simulink model "VehRT_211219"  (R2019b)
settings: Solver=ode5  StartTime=0.0  StopTime=Inf  FixedStep=Ts  RelTol=1e-3  EnableMultiTasking=on
InitFcn:
  | VehRT_Init_211219;
  | Ts=0.0005;
values from neighbouring files (symbols this model uses):
  damping_p = 0.113    [VehRT_Init_211219.m]
  Ff_ab_p = 0.41    [VehRT_Init_211219.m]
  Ff_c_p = 0.4    [VehRT_Init_211219.m]
  friction_enable = 1    [VehRT_Init_211219.m]
  sigma0_p = 200    [VehRT_Init_211219.m]
  sigma1_p = (200)^0.5    (= 14.1421356237)    [VehRT_Init_211219.m]
  td = 0.01    [VehRT_Init_211219.m]
  theta_sb_p = 0.03    [VehRT_Init_211219.m]
undefined symbols (not defined in the file or in its folder): C, canChannel, D, DiscIntNeverNeededParam, g, IO306, Kf, Kr, Lf, Lr, M, magnitude, sigma, trajectory_x11_, trajectory_x12_, trajectory_x13_, trajectory_x14_, trajectory_x15_, trajectory_x16_, trajectory_x17_, trajectory_x21_, trajectory_x22_, trajectory_x23_, trajectory_x24_, trajectory_x25_, trajectory_x26_, trajectory_x27_, trajectory_y11_, trajectory_y12_, trajectory_y13_, trajectory_y14_, trajectory_y15_, trajectory_y16_, trajectory_y17_, trajectory_y21_, trajectory_y22_, trajectory_y23_, trajectory_y24_, trajectory_y25_, trajectory_y26_, trajectory_y27_, zeta
libraries: canmsglib x31, speedgoatlib_IO612 x20, slrtlib x15, simulink x5, speedgoatlib_IO133 x3, xpcutilitieslib x2, canlib x2, xpcrtudplib x2, speedgoatlib_fpga x1, speedgoatlib_fpga_dio x1, autolibshared x1, speedgoatlib_fpga_quadrature x1
(part 1 of 4)
settings Model: SimulationMode=external  Creator=CECLAB  LastModifiedBy=CECLAB
settings SolverCC: ConcurrentTasks=on  AutoInsertRateTranBlk=on  InsertRTBMode=Never (minimum delay)
settings DataIOCC: SaveFormat=StructureWithTime  SaveOutput=off  SignalLogging=off  DSMLogging=off  ReturnWorkspaceOutputs=off
settings OptimizationCC: BlockReduction=off  OptimizeBlockIOStorage=off  BufferReuse=off  GlobalBufferReuse=off  ExpressionFolding=off  LocalBlockOutputs=off  OptimizeDataStoreBuffers=off  BusAssignmentInplaceUpdate=off
settings DebuggingCC: ArithmeticOperatorsInVariantConditions=warning
settings HardwareCC: ProdBitPerPointer=32  ProdBitPerSizeT=32  ProdBitPerPtrDiffT=32  ProdLargestAtomicFloat=None  ProdWordSize=32  ProdLongLongMode=on  ProdHWDeviceType=Generic->32-bit x86 compatible
settings SFSimCC: SimUseLocalCustomCode=off  CustomCodeUndefinedFunction=UseInterfaceOnly
settings RTWCC: Description=Simulink Real-Time  SystemTargetFile=slrt.tlc  TemplateMakefile=slrt_default_tmf  RTWUseLocalCustomCode=off  CodeExecutionProfiling=on  RTWCompilerOptimization=on
settings SimulinkRealTimeCC: SupportVariableSizeSignals=on  PreserveStateflowLocalDataDimensions=off  RL32LogTETModifier=off  xPCConcurrentTasks=on

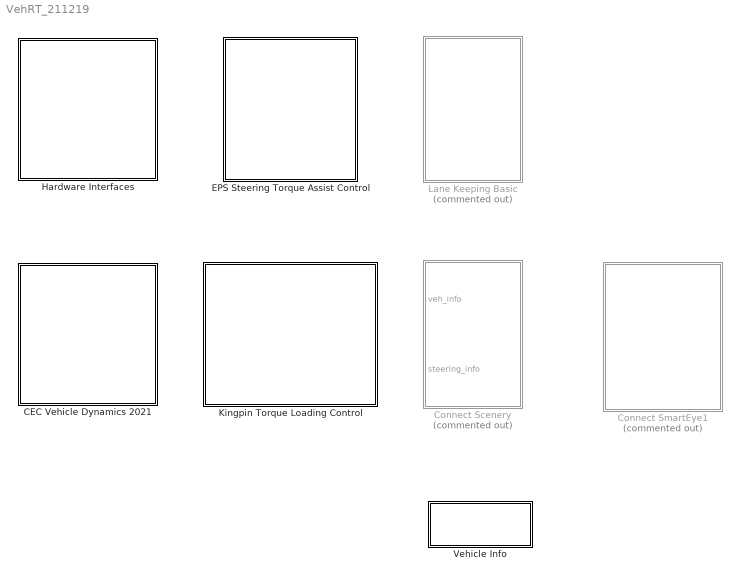
== system VehRT_211219 ==
  CEC Vehicle Dynamics 2021 : Subsystem
  Connect Scenery : Subsystem  Commented=on
  Connect SmartEye1 : Subsystem  Commented=on
  EPS Steering Torque Assist Control : Subsystem
  Hardware Interfaces : Subsystem
  Kingpin Torque Loading Control : Subsystem
  Lane Keeping Basic : Subsystem  Commented=on
  Vehicle Info : Subsystem

== system VehRT_211219/CEC Vehicle Dynamics 2021 ==
  note: CEC Vehicle Dynamics 2021
  Bus Selector : BusSelector  OutputSignals=str_Mpinion,veh_Vx
  CEC Vehicle Model 2021 : Subsystem  SystemSampleTime=0.001
      mask Display:
      | pos = get_param(gcb, 'Position');
      | width = pos(3) - pos(1);
      | height = pos(4) - pos(2);
      | p = min(width, height);
      | qx = (width-p)/2;
      | qy = (height-p)/2;
      | plt_body = [0.504672897196262,0.795560747663551;0.586448598130841,0.870327102803738;0.626168224299065,0.882009345794393;0.684579439252337,0.877336448598131;0.745327102803738,0.842289719626168;0.817757009345794,0.786214953271028;0.871495327102804,0.706775700934579;0.887850467289720,0.676401869158879;0.890186915887851,0.629672897196262;0.878504672897196,0.580607476635514;0.869158878504673,0.564252336448598;0.773364485981309,0.473130841121495;0.778037383177570,0.421728971962617;0.775700934579439,0.407710280373832;0.761682242990654,0.393691588785047;0.747663551401869,0.393691588785047;0.735981308411215,0.431074766355140;0.455607476635514,0.155373831775701;0.401869158878505,0.113317757009346;0.352803738317757,0.0852803738317758;0.313084112149533,0.0876168224299065;0.273364485981308,0.0992990654205608;0.207943925233645,0.160046728971963;0.149532710280374,0.220794392523365;0.107476635514019,0.267523364485981;0.0957943925233645,0.318925233644860;0.0981308411214953,0.358644859813084;0.121495327102804,0.400700934579439;0.441588785046729,0.730140186915888;0.404205607476636,0.732476635514019;0.397196261682243,0.741822429906542;0.401869158878505,0.760514018691589;0.422897196261682,0.769859813084112;0.453271028037383,0.762850467289720;0.478971962616822,0.762850467289720;0.504672897196262,0.795560747663551];
      | plt_body2 = [0.492990654205608,0.744158878504673;0.530373831775701,0.718457943925234;0.593457943925234,0.669392523364486;0.637850467289720,0.622663551401869;0.689252336448598,0.568925233644860;0.719626168224299,0.526869158878505;0.747663551401869,0.484813084112150;0.630841121495327,0.445093457943925;0.457943925233645,0.620327102803738;0.455607476635514,0.632009345794393;0.492990654205608,0.744158878504673];
      | plt_body3 = [0.635514018691589,0.424065420560748;0.740654205607477,0.461448598130841;0.448598130841122,0.176401869158878;0.469626168224299,0.255841121495327;0.635514018691589,0.424065420560748];
      | plt_body4 = [0.271028037383178,0.445093457943925;0.450934579439252,0.265186915887851;0.432242990654206,0.176401869158878;0.429906542056075,0.174065420560748;0.348130841121495,0.244158878504673;0.250000000000000,0.342289719626168;0.179906542056075,0.421728971962617;0.184579439252337,0.424065420560748;0.271028037383178,0.445093457943925]; %;0.186915887850467,0.447429906542056
      | plt_body5 = [0.266355140186916,0.463785046728972;0.184579439252337,0.445093457943925;0.469626168224299,0.727803738317757;0.432242990654206,0.620327102803738;0.266355140186916,0.463785046728972];
      | plt_body6 = [0.600467289719626,0.858644859813084;0.635514018691589,0.870327102803738;0.661214953271028,0.865654205607477;0.647196261682243,0.851635514018692;0.619158878504673,0.849299065420561;0.600467289719626,0.858644859813084];
      | plt_body7 = [0.866822429906542,0.596962616822430;0.857476635514019,0.610981308411215;0.862149532710280,0.636682242990654;0.871495327102804,0.655373831775701;0.871495327102804,0.657710280373832;0.876168224299065,0.632009345794393;0.871495327102804,0.594626168224299;0.866822429906542,0.596962616822430];
      | plt_body8 = [0.630841121495327,0.258177570093458;0.700934579439252,0.274532710280374;0.703271028037383,0.239485981308411;0.651869158878505,0.237149532710280;0.651869158878505,0.157710280373832;0.698598130841122,0.141355140186916;0.700934579439252,0.108644859813084;0.628504672897196,0.141355140186916;0.630841121495327,0.258177570093458];
      | plt_body9 = [0.710280373831776,0.272196261682243;0.707943925233645,0.113317757009346;0.785046728971963,0.132009345794393;0.785046728971963,0.155373831775701;0.742990654205608,0.150700934579439;0.740654205607477,0.178738317757009;0.785046728971963,0.185747663551402;0.787383177570094,0.206775700934579;0.742990654205608,0.209112149532710;0.740654205607477,0.241822429906542;0.785046728971963,0.234813084112150;0.785046728971963,0.260514018691589;0.710280373831776,0.272196261682243];
      | plt_body10 = [0.794392523364486,0.260514018691589;0.796728971962617,0.129672897196262;0.880841121495327,0.110981308411215;0.880841121495327,0.146028037383178;0.822429906542056,0.155373831775701;0.820093457943925,0.237149532710280;0.878504672897196,0.244158878504673;0.878504672897196,0.276869158878505;0.794392523364486,0.260514018691589];
      | plot([0,1,1,0]*width,[0,0,1,1]*height)
      | plot(plt_body(:,1)*p+qx,plt_body(:,2)*p+qy);
      | plot(plt_body2(:,1)*p+qx,plt_body2(:,2)*p+qy);
      | plot(plt_body3(:,1)*p+qx,plt_body3(:,2)*p+qy);
      | plot(plt_body4(:,1)*p+qx,plt_body4(:,2)*p+qy);
      | plot(plt_body5(:,1)*p+qx,plt_body5(:,2)*p+qy);
      | plot(plt_body6(:,1)*p+qx,plt_body6(:,2)*p+qy);
      | plot(plt_body7(:,1)*p+qx,plt_body7(:,2)*p+qy);
      | plot(plt_body8(:,1)*p+qx,plt_body8(:,2)*p+qy);
      | plot(plt_body9(:,1)*p+qx,plt_body9(:,2)*p+qy);
      | plot(plt_body10(:,1)*p+qx,plt_body10(:,2)*p+qy);
  Gain : Gain  Gain=0.01
  Gain1 : Gain  Gain=0.01
  Reset with Clutch : Subsystem
  manual_driving : Constant  Value=0
  mu_test : Subsystem
  zero_speed : Constant  Value=0
  tag scope: Veh_info=global, Vehicle_speed=global, pinion_torque=global
  wires:
  [pinion_angle] -> CEC Vehicle Model 2021/1(sta)
  [pedal_acc] -> Gain/1
  [pedal_brk] -> Gain1/1
  mu_test/1(mus) -> CEC Vehicle Model 2021/4(mu_road)
  zero_speed/1 -> CEC Vehicle Model 2021/5(spd_target)
  manual_driving/1 -> CEC Vehicle Model 2021/6(acc_mode)
  Reset with Clutch/1(rst) -> CEC Vehicle Model 2021/7(reset)
  CEC Vehicle Model 2021/1(Info) -> Bus Selector/1, [Veh_info]
  Bus Selector/1 -> [pinion_torque]  "<str_Mpinion>"
  Bus Selector/2 -> [Vehicle_speed]  "<veh_Vx>"
  Gain1/1 -> CEC Vehicle Model 2021/3(brk_m)
  Gain/1 -> CEC Vehicle Model 2021/2(thr_m)

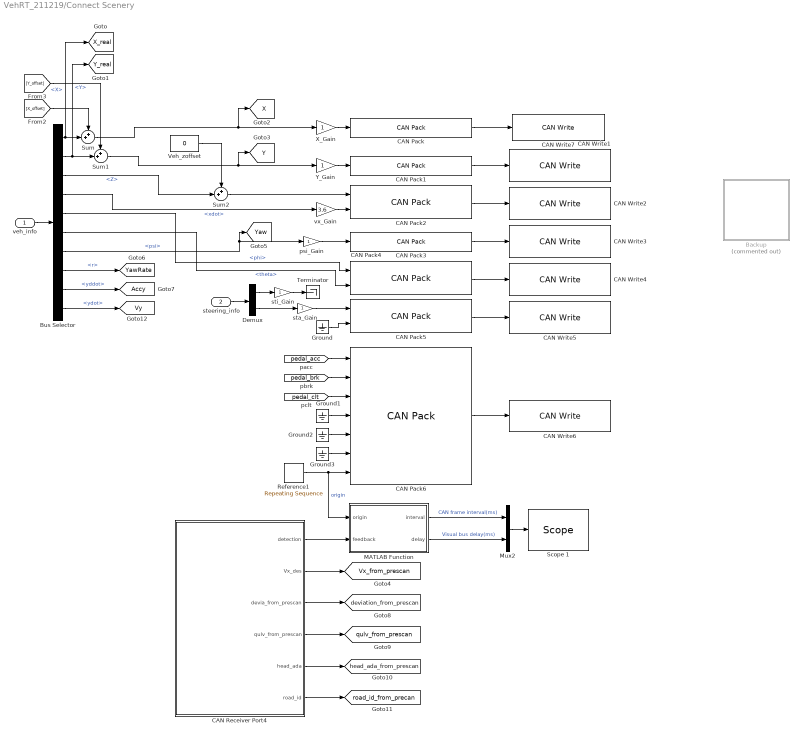
== system VehRT_211219/Connect Scenery ==
  veh_info : Inport
  steering_info : Inport  Port=2
  Backup : Subsystem  Commented=on
  Bus Selector : BusSelector  OutputSignals=InertFrm.Cg.Disp.X,InertFrm.Cg.Disp.Y,InertFrm.Cg.Disp.Z,BdyFrm.Cg.Vel.xdot,InertFrm.Cg.Ang.phi,InertFrm.Cg.Ang.theta,InertFrm.Cg.Ang.psi,BdyFrm.Cg.AngVel.r,BdyFrm.Cg.Acc.yddot,BdyFrm.Cg.Vel.ydot
  CAN Pack : canmsglib/CAN Pack  MsgList=(none)  MsgName=CAN Msg  MsgIDType=Standard (11-bit identifier)  MsgIdentifier=100  MsgLength=8  Remote=off  ApplyMinMax=off  BusOutput=off  SignalInfo={ 'x', '0', '64', 'LE', 'double', 'Standard', '0', '1', '0', '-Inf', 'Inf' }
      settings: SourceProductName=Vehicle Network Toolbox  SourceProductBaseCode=VN  DataFormat=manually specified signals
  CAN Pack1 : canmsglib/CAN Pack  MsgList=(none)  MsgName=CAN Msg  MsgIDType=Standard (11-bit identifier)  MsgIdentifier=101  MsgLength=8  Remote=off  ApplyMinMax=off  BusOutput=off  SignalInfo={ 'y', '0', '64', 'LE', 'double', 'Standard', '0', '1', '0', '-Inf', 'Inf' }
      settings: SourceProductName=Vehicle Network Toolbox  SourceProductBaseCode=VN  DataFormat=manually specified signals
  CAN Pack2 : canmsglib/CAN Pack  MsgList=(none)  MsgName=CAN Msg  MsgIDType=Standard (11-bit identifier)  MsgIdentifier=102  MsgLength=8  Remote=off  ApplyMinMax=off  BusOutput=off  SignalInfo={ 'z', '0', '32', 'LE', 'single', 'Standard', '0', '1', '0', '-Inf', 'Inf'; 'vx', '32', '32', 'LE', 'single', 'Standard', '0', '1', '0', '-Inf', 'Inf' }
      settings: SourceProductName=Vehicle Network Toolbox  SourceProductBaseCode=VN  DataFormat=manually specified signals
  CAN Pack3 : canmsglib/CAN Pack  MsgList=(none)  MsgName=CAN Msg  MsgIDType=Standard (11-bit identifier)  MsgIdentifier=103  MsgLength=8  Remote=off  ApplyMinMax=off  BusOutput=off  SignalInfo={ 'yaw', '0', '64', 'LE', 'double', 'Standard', '0', '1', '0', '-Inf', 'Inf' }
      settings: SourceProductName=Vehicle Network Toolbox  SourceProductBaseCode=VN  DataFormat=manually specified signals
  CAN Pack4 : canmsglib/CAN Pack  MsgList=(none)  MsgName=CAN Msg  MsgIDType=Standard (11-bit identifier)  MsgIdentifier=104  MsgLength=8  Remote=off  ApplyMinMax=off  BusOutput=off  SignalInfo={ 'roll', '0', '32', 'LE', 'single', 'Standard', '0', '1', '0', '-Inf', 'Inf'; 'pitch', '32', '32', 'LE', 'single', 'Standard', '0', '1', '0', '-Inf', 'Inf' }
      settings: SourceProductName=Vehicle Network Toolbox  SourceProductBaseCode=VN  DataFormat=manually specified signals
  CAN Pack5 : canmsglib/CAN Pack  MsgList=(none)  MsgName=CAN Msg  MsgIDType=Standard (11-bit identifier)  MsgIdentifier=105  MsgLength=8  Remote=off  ApplyMinMax=off  BusOutput=off  SignalInfo={ 'sta', '0', '32', 'LE', 'single', 'Standard', '0', '1', '0', '-Inf', 'Inf'; 'reserved', '32', '32', 'LE', 'single', 'Standard', '0', '1', '0', '-Inf', 'Inf' }
      settings: SourceProductName=Vehicle Network Toolbox  SourceProductBaseCode=VN  DataFormat=manually specified signals
  CAN Pack6 : canmsglib/CAN Pack  MsgList=(none)  MsgName=CAN Msg  MsgIDType=Standard (11-bit identifier)  MsgIdentifier=106  MsgLength=8  Remote=off  ApplyMinMax=off  BusOutput=off  SignalInfo={ 'pedal_acc', '0', '8', 'LE', 'unsigned', 'Standard', '0', '1', '0', '-Inf', 'Inf'; 'pedal_brk', '8', '8', 'LE', 'unsigned', 'Standard', '0', '1', '0', '-Inf', 'Inf'; 'pedal_clt', '16', '8', 'LE', 'unsigned', 'Standard', '0', '1', '0', '-Inf', 'Inf'; 'sw1', '24', '8', 'LE', 'unsigned', 'Standard', '0', '1', '0', '-Inf', 'Inf'; 'sw2', '32', '8', 'LE', 'unsigned', 'Standard', '0', '1', '0', '-Inf', 'Inf'; 'sw3', '40', '8', 'LE', 'unsigned', 'Standard', '0', '1', '0', '-Inf', 'Inf'; 'test', '48', '16', 'LE', 'unsigned', 'Standard', '0', '1', '0', '-Inf', 'Inf' }
      settings: SourceProductName=Vehicle Network Toolbox  SourceProductBaseCode=VN  DataFormat=manually specified signals
  CAN Receiver Port4 : Subsystem  TreatAsAtomicUnit=on
  CAN Write{1..7} (7 alike) : speedgoatlib_IO612/CAN Write  id=1  sampleTime=0.005  portSelection=2  messageType=CAN  enaStatusPort=off  protl=IO612  ptIdx=1  isFDMod=0
      settings: SourceProductName=Simulink Real-Time: Speedgoat Library
  Demux : Demux  Outputs=2
  Ground{,1..3} (4 alike) : Ground
  MATLAB Function : MATLAB Function  TreatAsAtomicUnit=on  SystemSampleTime=0.001
  Mux2 : Mux  Inputs=2
  Reference1 : simulink/Sources/Repeating Sequence  rep_seq_t=[0 2]  rep_seq_y=[0 65535]
  Scope 1 : slrtlib/Displays and Logging/Scope   scopeno=14  scopetype=Target  autostart=on  viewmode=Graphical sliding  formatstr='%15.6f'  grid=on  ylimits=[0,200]  nosamples=4000  noprepostsamples=0  interleave=1  triggermode=FreeRun  triggersignal=1  trigsignalfromport=off  triggerlevel=0.0  triggerslope=Either  triggerscope=1  triggersample=0  filename=data.dat  mode=Lazy  writesize=512  autorestart=off  dynamicfilemode=off  maxwritefilesize=512*1024^2
  Sum : Sum  Inputs=++|
  Sum1 : Sum  Inputs=++|
  Sum2 : Sum  Inputs=++|
  Terminator : Terminator
  Veh_zoffset : Constant  Value=0
  X_Gain : Gain
  Y_Gain : Gain
  psi_Gain : Gain
  sta_Gain : Gain
  sti_Gain : Gain
  "vx_Gain " : Gain  Gain=3.6
  tag scope: Accy=global, Vx_from_prescan=global, Vy=global, X=global, X_real=global, Y=global, Y_real=global, Yaw=global, YawRate=global, deviation_from_prescan=global, head_ada_from_prescan=global, qulv_from_prescan=global, road_id_from_precan=global
  wires:
  sta_Gain/1 -> CAN Pack5/1
  Demux/1 -> sti_Gain/1
  sti_Gain/1 -> Terminator/1
  Bus Selector/7 -> [Yaw], psi_Gain/1  "<psi>"
  Bus Selector/1 -> [X_real], Sum/2  "<X>"
  Bus Selector/3 -> Sum2/2  "<Z>"
  Bus Selector/2 -> [Y_real], Sum1/2  "<Y>"
  veh_info/1 -> Bus Selector/1
  steering_info/1 -> Demux/1
  Demux/2 -> sta_Gain/1
  MATLAB Function/2(delay) -> Mux2/2  "Visual bus delay(ms)"
  Mux2/1 -> Scope 1/1
  MATLAB Function/1(interval) -> Mux2/1  "CAN frame interval(ms)"
  Sum/1 -> [X], X_Gain/1
  Sum1/1 -> [Y], Y_Gain/1
  [X_offset] -> Sum/1
  [Y_offset] -> Sum1/1
  Bus Selector/4 -> "vx_Gain "/1  "<xdot>"
  "vx_Gain "/1 -> CAN Pack2/2
  Bus Selector/5 -> CAN Pack4/1  "<phi>"
  Bus Selector/6 -> CAN Pack4/2  "<theta>"
  X_Gain/1 -> CAN Pack/1
  Y_Gain/1 -> CAN Pack1/1
  Ground/1 -> CAN Pack5/2
  [pedal_acc] -> CAN Pack6/1
  [pedal_brk] -> CAN Pack6/2
  [pedal_clt] -> CAN Pack6/3
  Ground1/1 -> CAN Pack6/4
  Ground2/1 -> CAN Pack6/5
  Ground3/1 -> CAN Pack6/6
  Reference1/1 -> CAN Pack6/7, MATLAB Function/1(origin)  "origin"
  CAN Receiver Port4/1(detection) -> MATLAB Function/2(feedback)
  CAN Receiver Port4/2(Vx_des) -> [Vx_from_prescan]
  Sum2/1 -> CAN Pack2/1
  Veh_zoffset/1 -> Sum2/1
  Bus Selector/8 -> [YawRate]  "<r>"
  Bus Selector/9 -> [Accy]  "<yddot>"
  CAN Receiver Port4/3(devia_from_prescan) -> [deviation_from_prescan]
  CAN Receiver Port4/4(qulv_from_prescan) -> [qulv_from_prescan]
  CAN Receiver Port4/5(head_ada) -> [head_ada_from_prescan]
  psi_Gain/1 -> CAN Pack3/1
  CAN Receiver Port4/6(road_id) -> [road_id_from_precan]
  Bus Selector/10 -> [Vy]  "<ydot>"
  CAN Pack/1 -> CAN Write7/1
  CAN Pack6/1 -> CAN Write6/1
  CAN Pack1/1 -> CAN Write1/1
  CAN Pack2/1 -> CAN Write2/1
  CAN Pack3/1 -> CAN Write3/1
  CAN Pack4/1 -> CAN Write4/1
  CAN Pack5/1 -> CAN Write5/1

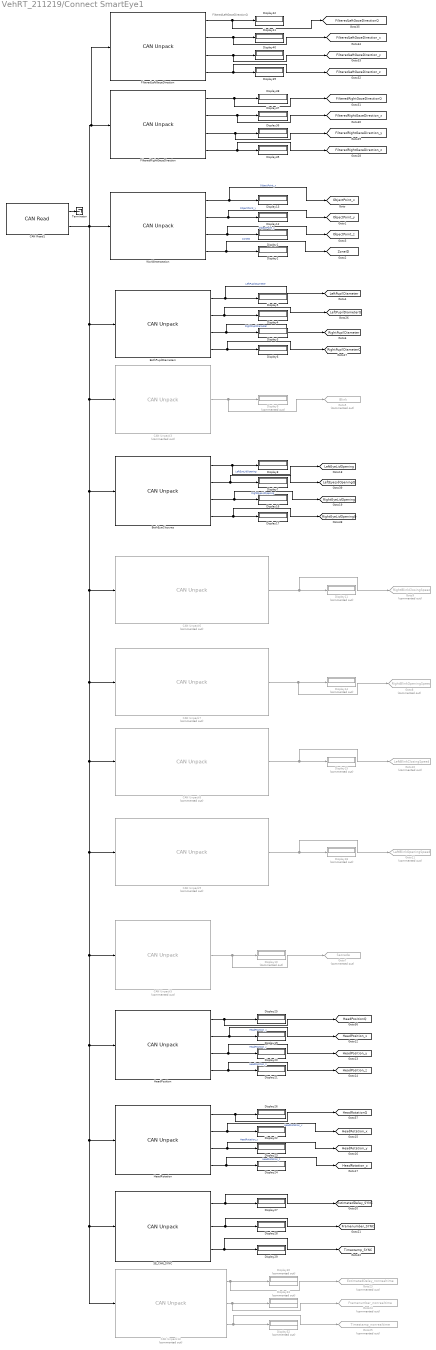
== system VehRT_211219/Connect SmartEye1 ==
  note: FilteredLeftGazeDirectionQ
  BothEyeClosures : canmsglib/CAN Unpack  CANdbFile=D:\Simulink\chenjiachen\realtime\smarteye.dbc  MsgList=SE_CAN_BOTHEYECLOSURES  MsgName=SE_CAN_BOTHEYECLOSURES  MsgIDType=Standard (11-bit identifier)  MsgIdentifier=1032  MsgLength=8  SignalInfo={'LeftEyeLidOpening','0','16','LE','signed','Standard','0','0.1','0','-3276.8','3276.7';'LeftEyeLidOpeningQ','16','16','LE','unsigned','Standard','0','0.0001','0','0','1';'RightEyeLidOpening','32','16','LE','signed','Standard','0','0.1','0','-3276.8','3276.7';'RightEyeLidOpeningQ','48','16','LE','unsigned','Standard','0','0.0001','0','0','1'}  IDPort=off  TimestampPort=off  ErrorPort=off  RemotePort=off  LengthPort=off  StatusPort=off  ApplyMinMax=off
      settings: SourceProductName=Simulink Real-Time  DataFormat=CANdb specified signals
  BothPupilDiameters : canmsglib/CAN Unpack  CANdbFile=D:\Simulink\chenjiachen\realtime\smarteye.dbc  MsgList=SE_CAN_BOTHPUPILDIAMETERS  MsgName=SE_CAN_BOTHPUPILDIAMETERS  MsgIDType=Standard (11-bit identifier)  MsgIdentifier=1034  MsgLength=8  SignalInfo={'LeftPupilDiameter','0','16','LE','signed','Standard','0','0.1','0','-3276.8','3276.7';'LeftPupilDiameterQ','16','16','LE','unsigned','Standard','0','0.0001','0','0','1';'RightPupilDiameter','32','16','LE','signed','Standard','0','0.1','0','-3276.8','3276.7';'RightPupilDiameterQ','48','16','LE','unsigned','Standard','0','0.0001','0','0','1'}  IDPort=off  TimestampPort=off  ErrorPort=off  RemotePort=off  LengthPort=off  StatusPort=off  ApplyMinMax=off
      settings: SourceProductName=Simulink Real-Time  DataFormat=CANdb specified signals
  CAN Read1 : speedgoatlib_IO612/CAN Read  id=1  sampleTime=-1  portSelection=3  messageType=CAN  protl=IO612  ptIdx=2  isFDMod=0
      settings: SourceProductName=Simulink Real-Time: Speedgoat Library
  CAN Unpack13 : canmsglib/CAN Unpack  Commented=on  CANdbFile=D:\Simulink\chenjiachen\realtime\smarteye.dbc  MsgList=SE_CAN_SYNCH_NON_REALTIME  MsgName=SE_CAN_SYNCH_NON_REALTIME  MsgIDType=Standard (11-bit identifier)  MsgIdentifier=1040  MsgLength=8  SignalInfo={'EstimatedDelay','48','16','LE','unsigned','Standard','0','0.1','0','0','6553.5';'Framenumber','0','32','LE','unsigned','Standard','0','1','0','0','4294967295';'Timestamp','32','16','LE','unsigned','Standard','0','0.1','0','0','6553.5'}  IDPort=off  TimestampPort=off  ErrorPort=off  RemotePort=off  LengthPort=off  StatusPort=off  ApplyMinMax=off
      settings: SourceProductName=Simulink Real-Time  DataFormat=CANdb specified signals
  CAN Unpack3 : canmsglib/CAN Unpack  Commented=on  CANdbFile=D:\Simulink\chenjiachen\realtime\smarteye.dbc  MsgList=SE_CAN_BLINK  MsgName=SE_CAN_BLINK  MsgIDType=Standard (11-bit identifier)  MsgIdentifier=1042  MsgLength=4  SignalInfo={'Blink','0','32','LE','unsigned','Standard','0','1','0','0','1'}  IDPort=off  TimestampPort=off  ErrorPort=off  RemotePort=off  LengthPort=off  StatusPort=off  ApplyMinMax=off
      settings: SourceProductName=Simulink Real-Time  DataFormat=CANdb specified signals
  CAN Unpack5 : canmsglib/CAN Unpack  Commented=on  CANdbFile=D:\Simulink\chenjiachen\realtime\smarteye.dbc  MsgList=SE_CAN_SACCADE  MsgName=SE_CAN_SACCADE  MsgIDType=Standard (11-bit identifier)  MsgIdentifier=1043  MsgLength=4  SignalInfo={'Saccade','0','32','LE','unsigned','Standard','0','1','0','0','1'}  IDPort=off  TimestampPort=off  ErrorPort=off  RemotePort=off  LengthPort=off  StatusPort=off  ApplyMinMax=off
      settings: SourceProductName=Simulink Real-Time  DataFormat=CANdb specified signals
  CAN Unpack6 : canmsglib/CAN Unpack  Commented=on  CANdbFile=D:\Simulink\chenjiachen\realtime\smarteye.dbc  MsgList=SE_CAN_RIGHTBLINKCLOSINGSPEED  MsgName=SE_CAN_RIGHTBLINKCLOSINGSPEED  MsgIDType=Standard (11-bit identifier)  MsgIdentifier=1052  MsgLength=2  SignalInfo={'RightBlinkClosingSpeed','0','16','LE','signed','Standard','0','0.0001','0','-3.2768','3.2767'}  IDPort=off  TimestampPort=off  ErrorPort=off  RemotePort=off  LengthPort=off  StatusPort=off  ApplyMinMax=off
      settings: SourceProductName=Simulink Real-Time  DataFormat=CANdb specified signals
  CAN Unpack7 : canmsglib/CAN Unpack  Commented=on  CANdbFile=D:\Simulink\chenjiachen\realtime\smarteye.dbc  MsgList=SE_CAN_RIGHTBLINKOPENINGSPEED  MsgName=SE_CAN_RIGHTBLINKOPENINGSPEED  MsgIDType=Standard (11-bit identifier)  MsgIdentifier=1055  MsgLength=2  SignalInfo={'RightBlinkOpeningSpeed','0','16','LE','signed','Standard','0','0.0001','0','-3.2768','3.2767'}  IDPort=off  TimestampPort=off  ErrorPort=off  RemotePort=off  LengthPort=off  StatusPort=off  ApplyMinMax=off
      settings: SourceProductName=Simulink Real-Time  DataFormat=CANdb specified signals
  CAN Unpack8 : canmsglib/CAN Unpack  Commented=on  CANdbFile=D:\Simulink\chenjiachen\realtime\smarteye.dbc  MsgList=SE_CAN_LEFTBLINKCLOSINGSPEED  MsgName=SE_CAN_LEFTBLINKCLOSINGSPEED  MsgIDType=Standard (11-bit identifier)  MsgIdentifier=1046  MsgLength=2  SignalInfo={'LeftBlinkClosingSpeed','0','16','LE','signed','Standard','0','0.0001','0','-3.2768','3.2767'}  IDPort=off  TimestampPort=off  ErrorPort=off  RemotePort=off  LengthPort=off  StatusPort=off  ApplyMinMax=off
      settings: SourceProductName=Simulink Real-Time  DataFormat=CANdb specified signals
  CAN Unpack9 : canmsglib/CAN Unpack  Commented=on  CANdbFile=D:\Simulink\chenjiachen\realtime\smarteye.dbc  MsgList=SE_CAN_LEFTBLINKOPENINGSPEED  MsgName=SE_CAN_LEFTBLINKOPENINGSPEED  MsgIDType=Standard (11-bit identifier)  MsgIdentifier=1049  MsgLength=2  SignalInfo={'LeftBlinkOpeningSpeed','0','16','LE','signed','Standard','0','0.0001','0','-3.2768','3.2767'}  IDPort=off  TimestampPort=off  ErrorPort=off  RemotePort=off  LengthPort=off  StatusPort=off  ApplyMinMax=off
      settings: SourceProductName=Simulink Real-Time  DataFormat=CANdb specified signals
  Display{1..8,12..13,16..17,19..29,35..42} (31 alike) : Display
  Display{9..11,14..15,18,30,32..33} (9 alike) : Display  Commented=on
  FilteredLeftGazeDirection : canmsglib/CAN Unpack  CANdbFile=D:\Simulink\chenjiachen\realtime\smarteye.dbc  MsgList=SE_CAN_FILTEREDLEFTGAZEDIRECTION  MsgName=SE_CAN_FILTEREDLEFTGAZEDIRECTION  MsgIDType=Standard (11-bit identifier)  MsgIdentifier=1038  MsgLength=8  SignalInfo={'FilteredLeftGazeDirectionQ','48','16','LE','unsigned','Standard','0','0.0001','0','0','1';'FilteredLeftGazeDirection_x','0','16','LE','signed','Standard','0','0.0001','0','-1','1';'FilteredLeftGazeDirection_y','16','16','LE','signed','Standard','0','0.0001','0','-1','1';'FilteredLeftGazeDirection_z','32','16','LE','signed','Standard','0','0.0001','0','-1','1'}  IDPort=off  TimestampPort=off  ErrorPort=off  RemotePort=off  LengthPort=off  StatusPort=off  ApplyMinMax=off
      settings: SourceProductName=Simulink Real-Time  DataFormat=CANdb specified signals
  FilteredRightGazeDirection : canmsglib/CAN Unpack  CANdbFile=D:\Simulink\chenjiachen\realtime\smarteye.dbc  MsgList=SE_CAN_FILTEREDRIGHTGAZEDIRECTION  MsgName=SE_CAN_FILTEREDRIGHTGAZEDIRECTION  MsgIDType=Standard (11-bit identifier)  MsgIdentifier=1039  MsgLength=8  SignalInfo={'FilteredRightGazeDirectionQ','48','16','LE','unsigned','Standard','0','0.0001','0','0','1';'FilteredRightGazeDirection_x','0','16','LE','signed','Standard','0','0.0001','0','-1','1';'FilteredRightGazeDirection_y','16','16','LE','signed','Standard','0','0.0001','0','-1','1';'FilteredRightGazeDirection_z','32','16','LE','signed','Standard','0','0.0001','0','-1','1'}  IDPort=off  TimestampPort=off  ErrorPort=off  RemotePort=off  LengthPort=off  StatusPort=off  ApplyMinMax=off
      settings: SourceProductName=Simulink Real-Time  DataFormat=CANdb specified signals
  Goto10 : Goto  Commented=on  GotoTag=LeftBlinkClosingSpeed  TagVisibility=global
  Goto11 : Goto  Commented=on  GotoTag=LeftBlinkOpeningSpeed  TagVisibility=global
  Goto23 : Goto  Commented=on  GotoTag=EstimatedDelay_nonrealtime  TagVisibility=global
  Goto24 : Goto  Commented=on  GotoTag=Framenumber_nonrealtime  TagVisibility=global
  Goto25 : Goto  Commented=on  GotoTag=Timestamp_nonrealtime  TagVisibility=global
  Goto5 : Goto  Commented=on  GotoTag=Blink  TagVisibility=global
  Goto7 : Goto  Commented=on  GotoTag=Saccade  TagVisibility=global
  Goto8 : Goto  Commented=on  GotoTag=RightBlinkOpeningSpeed  TagVisibility=global
  Goto9 : Goto  Commented=on  GotoTag=RightBlinkClosingSpeed  TagVisibility=global
  HeadPosition : canmsglib/CAN Unpack  CANdbFile=D:\Simulink\chenjiachen\realtime\smarteye.dbc  MsgList=SE_CAN_HEADPOSITION  MsgName=SE_CAN_HEADPOSITION  MsgIDType=Standard (11-bit identifier)  MsgIdentifier=1027  MsgLength=8  SignalInfo={'HeadPositionQ','48','16','LE','unsigned','Standard','0','0.0001','0','0','1';'HeadPosition_x','0','16','LE','signed','Standard','0','0.1','0','-3276.8','3276.7';'HeadPosition_y','16','16','LE','signed','Standard','0','0.1','0','-3276.8','3276.7';'HeadPosition_z','32','16','LE','signed','Standard','0','0.1','0','-3276.8','3276.7'}  IDPort=off  TimestampPort=off  ErrorPort=off  RemotePort=off  LengthPort=off  StatusPort=off  ApplyMinMax=off
      settings: SourceProductName=Simulink Real-Time  DataFormat=CANdb specified signals
  HeadRotation : canmsglib/CAN Unpack  CANdbFile=D:\Simulink\chenjiachen\realtime\smarteye.dbc  MsgList=SE_CAN_HEADROTATION  MsgName=SE_CAN_HEADROTATION  MsgIDType=Standard (11-bit identifier)  MsgIdentifier=1028  MsgLength=8  SignalInfo={'HeadRotationQ','48','16','LE','unsigned','Standard','0','0.0001','0','0','1';'HeadRotation_x','0','16','LE','signed','Standard','0','0.0001','0','-3.2768','3.2767';'HeadRotation_y','16','16','LE','signed','Standard','0','0.0001','0','-3.2768','3.2767';'HeadRotation_z','32','16','LE','signed','Standard','0','0.0001','0','-3.2768','3.2767'}  IDPort=off  TimestampPort=off  ErrorPort=off  RemotePort=off  LengthPort=off  StatusPort=off  ApplyMinMax=off
      settings: SourceProductName=Simulink Real-Time  DataFormat=CANdb specified signals
  SE_CAN_SYNC : canmsglib/CAN Unpack  CANdbFile=D:\Simulink\chenjiachen\realtime\smarteye.dbc  MsgList=SE_CAN_SYNC  MsgName=SE_CAN_SYNC  MsgIDType=Standard (11-bit identifier)  MsgIdentifier=1025  MsgLength=8  SignalInfo={'EstimatedDelay','48','16','LE','unsigned','Standard','0','0.1','0','0','6553.5';'Framenumber','0','32','LE','unsigned','Standard','0','1','0','0','4294967295';'Timestamp','32','16','LE','unsigned','Standard','0','0.1','0','0','6553.5'}  IDPort=off  TimestampPort=off  ErrorPort=off  RemotePort=off  LengthPort=off  StatusPort=off  ApplyMinMax=off
      settings: SourceProductName=Simulink Real-Time  DataFormat=CANdb specified signals
  Terminator : Terminator
  WorldIntersection : canmsglib/CAN Unpack  CANdbFile=D:\Simulink\chenjiachen\realtime\smarteye.dbc  MsgList=SE_CAN_WORLDINTERSECTION  MsgName=SE_CAN_WORLDINTERSECTION  MsgIDType=Standard (11-bit identifier)  MsgIdentifier=1036  MsgLength=8  SignalInfo={'ObjectPoint_x','16','16','LE','signed','Standard','0','0.1','0','-3276.8','3276.7';'ObjectPoint_y','32','16','LE','signed','Standard','0','0.1','0','-3276.8','3276.7';'ObjectPoint_z','48','16','LE','signed','Standard','0','0.1','0','-3276.8','3276.7';'ZoneID','0','16','LE','unsigned','Standard','0','1','0','0','65535'}  IDPort=off  TimestampPort=off  ErrorPort=off  RemotePort=off  LengthPort=off  StatusPort=off  ApplyMinMax=off
      settings: SourceProductName=Simulink Real-Time  DataFormat=CANdb specified signals
  tag scope: EstimatedDelay_SYNC=global, FilteredLeftGazeDirectionQ=global, FilteredLeftGazeDirection_x=global, FilteredLeftGazeDirection_y=global, FilteredLeftGazeDirection_z=global, FilteredRightGazeDirectionQ=global, FilteredRightGazeDirection_x=global, FilteredRightGazeDirection_y=global, FilteredRightGazeDirection_z=global, Framenumber_SYNC=global, HeadPositionQ=global, HeadPosition_x=global, HeadPosition_y=global, HeadPosition_z=global, HeadRotationQ=global, HeadRotation_x=global, HeadRotation_y=global, HeadRotation_z=global, LeftEyeLidOpening=global, LeftEyeLidOpeningQ=global, LeftPupilDiameter=global, LeftPupilDiameterQ=global, ObjectPoint_x=global, ObjectPoint_y=global, ObjectPoint_z=global, RightEyeLidOpening=global, RightEyeLidOpeningQ=global, RightPupilDiameter=global, RightPupilDiameterQ=global, Timestamp_SYNC=global, ZoneID=global
  wires:
  WorldIntersection/2 -> [ObjectPoint_y], Display12/1  "ObjectPoint_y"
  WorldIntersection/1 -> [ObjectPoint_x], Display13/1  "ObjectPoint_x"
  CAN Read1/2 -> FilteredLeftGazeDirection/1, FilteredRightGazeDirection/1, CAN Unpack9/1, CAN Unpack13/1, SE_CAN_SYNC/1, HeadRotation/1, HeadPosition/1, CAN Unpack5/1, CAN Unpack8/1, CAN Unpack7/1, CAN Unpack6/1, BothEyeClosures/1, CAN Unpack3/1, BothPupilDiameters/1, WorldIntersection/1
  WorldIntersection/4 -> [ZoneID], Display2/1  "ZoneID"
  WorldIntersection/3 -> [ObjectPoint_z], Display1/1  "ObjectPoint_z"
  BothPupilDiameters/1 -> [LeftPupilDiameter], Display5/1  "LeftPupilDiameter"
  BothPupilDiameters/2 -> [LeftPupilDiameterQ], Display4/1
  BothPupilDiameters/3 -> [RightPupilDiameter], Display3/1  "RightPupilDiameter"
  BothPupilDiameters/4 -> [RightPupilDiameterQ], Display6/1
  BothEyeClosures/2 -> [LeftEyeLidOpeningQ], Display7/1
  BothEyeClosures/1 -> [LeftEyeLidOpening], Display8/1  "LeftEyeLidOpening"
  CAN Unpack3/1 -> Goto5/1, Display9/1
  CAN Unpack5/1 -> Goto7/1, Display10/1
  BothEyeClosures/3 -> [RightEyeLidOpening], Display16/1  "RightEyeLidOpening"
  BothEyeClosures/4 -> [RightEyeLidOpeningQ], Display17/1
  CAN Unpack6/1 -> Goto9/1, Display11/1
  CAN Unpack7/1 -> Goto8/1, Display14/1
  CAN Unpack8/1 -> Display15/1, Goto10/1
  CAN Unpack9/1 -> Goto11/1, Display18/1
  HeadPosition/2 -> [HeadPosition_x], Display19/1  "HeadPosition_x"
  HeadPosition/3 -> [HeadPosition_y], Display20/1  "HeadPosition_y"
  HeadPosition/4 -> [HeadPosition_z], Display21/1  "HeadPosition_z"
  HeadRotation/2 -> [HeadRotation_x], Display22/1  "HeadRotation_x"
  HeadRotation/3 -> [HeadRotation_y], Display23/1  "HeadRotation_y"
  HeadRotation/4 -> [HeadRotation_z], Display24/1  "HeadRotation_z"
  HeadPosition/1 -> [HeadPositionQ], Display25/1
  HeadRotation/1 -> [HeadRotationQ], Display26/1
  SE_CAN_SYNC/1 -> [EstimatedDelay_SYNC], Display27/1
  SE_CAN_SYNC/2 -> [Framenumber_SYNC], Display28/1
  SE_CAN_SYNC/3 -> [Timestamp_SYNC], Display29/1
  CAN Unpack13/1 -> Goto23/1, Display30/1
  CAN Unpack13/2 -> Goto24/1, Display33/1
  CAN Unpack13/3 -> Goto25/1, Display32/1
  CAN Read1/1 -> Terminator/1
  FilteredRightGazeDirection/1 -> [FilteredRightGazeDirectionQ], Display38/1
  FilteredRightGazeDirection/2 -> [FilteredRightGazeDirection_x], Display37/1
  FilteredRightGazeDirection/3 -> [FilteredRightGazeDirection_y], Display36/1
  FilteredRightGazeDirection/4 -> [FilteredRightGazeDirection_z], Display35/1
  FilteredLeftGazeDirection/1 -> [FilteredLeftGazeDirectionQ], Display42/1
  FilteredLeftGazeDirection/2 -> [FilteredLeftGazeDirection_x], Display41/1
  FilteredLeftGazeDirection/3 -> [FilteredLeftGazeDirection_y], Display40/1
  FilteredLeftGazeDirection/4 -> [FilteredLeftGazeDirection_z], Display39/1

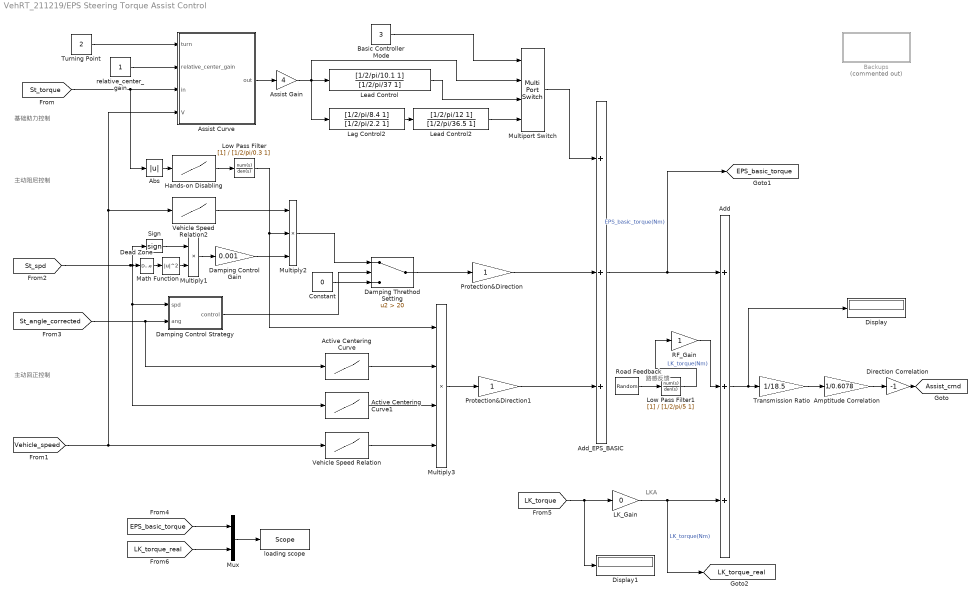
== system VehRT_211219/EPS Steering Torque Assist Control ==
  note: 主动阻尼控制
  note: 基础助力控制
  note: 主动回正控制
  note: 路感反馈
  note: LKA
  Abs : Abs
  Active Centering Curve : Lookup_n-D  NumberOfTableDimensions=1  BreakpointsForDimension1=[-90 -70 -50 -12 -3 0 3 12 50 70 90]  Table=[0 0 -1 -1 -0.15 0 0.15 1 1 0 0]  InternalRulePriority=Speed  RndMeth=Simplest  InputSameDT=on
  Active Centering Curve1 : Lookup_n-D  NumberOfTableDimensions=1  BreakpointsForDimension1=[-100 -60 -40 -20 -10 0 10 20 40 60 100]  Table=[0 0 0.1 0.8 1 1.1 1 0.8 0.1 0 0]  InternalRulePriority=Speed  RndMeth=Simplest  InputSameDT=on
  Add : Sum  Inputs=+++
  Add_EPS_BASIC : Sum  Inputs=+++
  Amptitude Correlation : Gain  Gain=1/0.6078
  Assist Curve : MATLAB Function  TreatAsAtomicUnit=on
  Assist Gain : Gain  Gain=4
  Backups : Subsystem  Commented=on
  Basic Controller Mode : Constant  Value=3
  Constant : Constant  Value=0
  Damping Control Gain : Gain  Gain=0.001
  Damping Control Strategy : MATLAB Function
  Damping Threthod Setting : Switch  Criteria=u2 > Threshold  Threshold=20
  Dead Zone : DeadZone  LowerValue=-20  UpperValue=20  SaturateOnIntegerOverflow=on
  Direction Correlation : Gain  Gain=-1
  Display : Display
  Display1 : Display
  Hands-on Disabling : Lookup_n-D  NumberOfTableDimensions=1  BreakpointsForDimension1=[0 0.6 1.5 2.7 5]  Table=[1 1 0.2 0 0 ]  InternalRulePriority=Speed  RndMeth=Simplest  InputSameDT=on
  LK_Gain : Gain  Gain=0
  Lag Control2 : TransferFcn  Numerator=[1/2/pi/8.4 1]  Denominator=[1/2/pi/2.2 1]
  Lead Control : TransferFcn  Numerator=[1/2/pi/10.1 1]  Denominator=[1/2/pi/37 1]
  Lead Control2 : TransferFcn  Numerator=[1/2/pi/12 1]  Denominator=[1/2/pi/36.5 1]
  Low Pass Filter : TransferFcn  Denominator=[1/2/pi/0.3 1]
  Low Pass Filter1 : TransferFcn  Denominator=[1/2/pi/5 1]
  Math Function : Math  Operator=magnitude^2  SaturateOnIntegerOverflow=on
  Multiply1 : Product
  Multiply2 : Product  Inputs=3
  Multiply3 : Product  Inputs=4
  Multiport Switch : MultiPortSwitch
  Mux : Mux  Inputs=2
  Protection&Direction : Gain
  Protection&Direction1 : Gain
  RF_Gain : Gain
  Road Feedback : RandomNumber  Variance=0.8
  Sign : Signum
  Transmission Ratio : Gain  Gain=1/18.5
  Turning Point : Constant  Value=2
  Vehicle Speed Relation : Lookup_n-D  NumberOfTableDimensions=1  BreakpointsForDimension1=[0 40 50 60 80 110 120]  Table=[3.5 3.5 1.1 0.4 0.2 0 0]  InternalRulePriority=Speed  RndMeth=Simplest  InputSameDT=on
  Vehicle Speed Relation2 : Lookup_n-D  NumberOfTableDimensions=1  BreakpointsForDimension1=[0 55 60 75 80 110 120 160 180]  Table=[0 0 0.1 0.3 1.0 1.9 2.6 3.8 4.0]  InternalRulePriority=Speed  RndMeth=Simplest  InputSameDT=on
  loading scope : slrtlib/Displays and Logging/Scope   scopeno=16  scopetype=Target  autostart=on  viewmode=Graphical rolling  formatstr='%15.6f'  grid=on  ylimits=[-30,30]  nosamples=1000  noprepostsamples=0  interleave=1  triggermode=FreeRun  triggersignal=1  trigsignalfromport=off  triggerlevel=0.0  triggerslope=Either  triggerscope=1  triggersample=0  filename=data.dat  mode=Lazy  writesize=512  autorestart=off  dynamicfilemode=off  maxwritefilesize=512*1024^2
  relative_center_gain : Constant
  tag scope: Assist_cmd=global, EPS_basic_torque=global, LK_torque_real=global
  wires:
  Assist Curve/1(out) -> Assist Gain/1
  Direction Correlation/1 -> [Assist_cmd]
  Assist Gain/1 -> Lag Control2/1, Lead Control/1, Multiport Switch/2
  [St_torque] -> Abs/1, Assist Curve/3(in)
  [St_angle_corrected] -> Damping Control Strategy/2(ang), Active Centering Curve/1
  Damping Threthod Setting/1 -> Protection&Direction/1
  Add/1 -> Display/1, Transmission Ratio/1
  Turning Point/1 -> Assist Curve/1(turn)
  [St_spd] -> Sign/1, Damping Control Strategy/1(spd), Active Centering Curve1/1, Dead Zone/1
  relative_center_gain/1 -> Assist Curve/2(relative_center_gain)
  Lag Control2/1 -> Lead Control2/1
  Amptitude Correlation/1 -> Direction Correlation/1
  Transmission Ratio/1 -> Amptitude Correlation/1
  Constant/1 -> Damping Threthod Setting/3
  Multiply3/1 -> Protection&Direction1/1
  Math Function/1 -> Multiply1/2
  Sign/1 -> Multiply1/1
  Multiply1/1 -> Damping Control Gain/1
  Abs/1 -> Hands-on Disabling/1
  Damping Control Strategy/1(control) -> Damping Threthod Setting/2
  Lead Control2/1 -> Multiport Switch/4
  Lead Control/1 -> Multiport Switch/3
  Basic Controller Mode/1 -> Multiport Switch/1
  Active Centering Curve/1 -> Multiply3/2
  Active Centering Curve1/1 -> Multiply3/3
  [Vehicle_speed] -> Assist Curve/4(V), Vehicle Speed Relation2/1, Vehicle Speed Relation/1
  Vehicle Speed Relation/1 -> Multiply3/4
  Low Pass Filter/1 -> Multiply3/1, Multiply2/2
  Multiply2/1 -> Damping Threthod Setting/1
  Damping Control Gain/1 -> Multiply2/3
  Hands-on Disabling/1 -> Low Pass Filter/1
  Road Feedback/1 -> Low Pass Filter1/1
  Low Pass Filter1/1 -> RF_Gain/1
  Vehicle Speed Relation2/1 -> Multiply2/1
  [LK_torque] -> Display1/1, LK_Gain/1
  LK_Gain/1 -> [LK_torque_real], Add/3  "LK_torque(Nm)"
  Add_EPS_BASIC/1 -> [EPS_basic_torque], Add/1  "EPS_basic_torque(Nm)"
  Protection&Direction1/1 -> Add_EPS_BASIC/3
  Protection&Direction/1 -> Add_EPS_BASIC/2
  Multiport Switch/1 -> Add_EPS_BASIC/1
  [EPS_basic_torque] -> Mux/1
  [LK_torque_real] -> Mux/2
  Mux/1 -> loading scope/1
  Dead Zone/1 -> Math Function/1
  RF_Gain/1 -> Add/2  "LK_torque(Nm)"

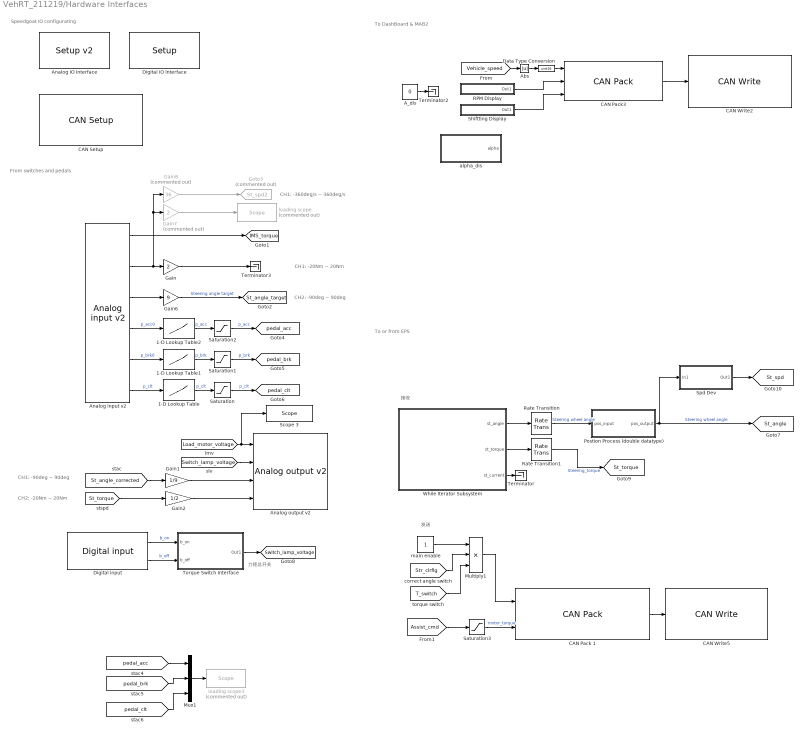
== system VehRT_211219/Hardware Interfaces ==
  note: To or from EPS
  note: From switches and pedals
  note: Speedgoat IO configurating
  note: To DashBoard & MAB2
  note: CH1: -90deg ~ 90deg
  note: CH2: -20Nm ~ 20Nm
  note: CH1: -20Nm ~ 20Nm
  note: CH2: -90deg ~ 90deg
  note: CH1: -360deg/s ~ 360deg/s
  note: 力矩总开关
  note: 接收
  note: 发送
  1-D Lookup Table : Lookup_n-D  NumberOfTableDimensions=1  BreakpointsForDimension1=[0.81,8.50]  Table=[100,0]  InternalRulePriority=Speed  RndMeth=Simplest  InputSameDT=on
  1-D Lookup Table1 : Lookup_n-D  NumberOfTableDimensions=1  BreakpointsForDimension1=[0.87,8.45]  Table=[100,0]  InternalRulePriority=Speed  RndMeth=Simplest  InputSameDT=on
  1-D Lookup Table2 : Lookup_n-D  NumberOfTableDimensions=1  BreakpointsForDimension1=[0.48,8.33]  Table=[100,0]  InternalRulePriority=Speed  RndMeth=Simplest  InputSameDT=on
  A_dis : Constant  Value=0
  Abs : Abs
  Analog IO Interface : speedgoatlib_IO133/Setup v2   parPciSlot=-1  parModuleId=1  parInterModuleSync=Independent  parConvClockBaseRate=20MHz  parConvClock1Divider=20000  parConvClock2Divider=20000  parFrameTriggerEnable=off  parFrameTriggerDivider=10  parConvClock1BaseRate=1  parConvClock2BaseRate=1  parFrameTriggerClock=1  parAdcChannels=[1 3 4 5 6 7]  parAdcRange1=+-10V  parAdcRange2=+-5V  parAdcVoltageRange=[2 1]  parAdcOversampling1=None  parAdcOversampling2=None  parAdcOversamplRate=[1 1]  parAdcAutoCorrection=on  parAdcContSampling=off  parAdcDmaEnable=off  parAdcDmaClock="Clock 1  (1 kHz)"  parAdcFrameSize_=100  parAdcSampleTime_=-1  parAdcActiveDmaDevices=[1 1]  parAdcFrameTriggerEnable=0  parAdcFrameSize=100  parAdcSampleTime=0.1  parDacChannels=[1 3 4 5]  parDacInitValues=0  parDacReset=1  parDacRange1=+-10V  parDacRange2=+-10V  parDacRange3=+-10V  parDacRange4=+-10V  parDacRange5=+-10V  parDacRange6=0-5V  parDacRange7=0-5V  parDacRange8=0-5V  parDacVoltageRange=[5 5 5 5 5 1 1 1]  parDacAutoCorrection=on  parDacSyncOut=on  parDacDmaEnable=off  parDacDmaLatency=Until next frame  parDacDmaClock="Clock 1  (1 kHz)"  parDacFrameSize_=100  parDacSampleTime_=-1  parDacActiveDmaDevices=[1 1]  parDacFrameTriggerEnable=0  parDacFrameSize=100  parDacSampleTime=0.1  parDoChannels=[1 2]  parDoInitValues=0  parDoReset=1  parDiChannels=[3 4]  parDiDebounceEnable=off  parDiDebounceTime=0  parDiDebounceValue=0  parDioPullRefFront=Pull-up 3.3V  parDioPullRefRear=Floating
      settings: SourceProductName=Simulink Real-Time: Speedgoat Library
  "Analog input v2 " : speedgoatlib_IO133/Analog input v2   parModuleId=1  parSampleTime=-1  parPciSlot=-1  parAdcChannels=[1 3 4 5 6 7]  parAdcVoltageRange=[2 1]  parAdcOversamplRate=[1 1]  parAdcContSampling=0  parAdcDmaEnable=0  parAdcActiveDmaDevices=[1 1]  parAdcFrameSize=100
      settings: SourceProductName=Simulink Real-Time: Speedgoat Library
  "Analog output v2 " : speedgoatlib_IO133/Analog output v2   parModuleId=1  parSampleTime=-1  parPciSlot=-1  parDacChannels=[1 3 4 5]  parDacVoltageRange=[5 5 5 5 5 1 1 1]  parDacInitValues=[0 0 0 0]  parDacReset=[1 1 1 1]  parDacSyncOut=1  parDacDmaEnable=0  parDacActiveDmaDevices=[1 1]  parDacDmaLatency=2  parDacFrameSize=100
      settings: SourceProductName=Simulink Real-Time: Speedgoat Library
  CAN Pack 1 : canmsglib/CAN Pack  CANdbFile=D:\Speedgoat\Simulink Test Model\EPS_Test_2018_0101.dbc  MsgList=MAB2EPS  MsgName=MAB2EPS  MsgIDType=Standard (11-bit identifier)  MsgIdentifier=2047  MsgLength=8  Remote=off  ApplyMinMax=off  BusOutput=off  SignalInfo={'DrivingMode','0','1','BE','unsigned','Standard','0','1','0','-Inf','Inf';'TorqueRequest','16','16','BE','signed','Standard','0','0.001','0','-Inf','Inf'}
      settings: SourceProductName=Simulink Real-Time  DataFormat=CANdb specified signals
  CAN Pack3 : canmsglib/CAN Pack  MsgList=(none)  MsgName=CAN Msg  MsgIDType=Standard (11-bit identifier)  MsgIdentifier=480  MsgLength=8  Remote=off  ApplyMinMax=off  BusOutput=off  SignalInfo={ 'vx_int', '0', '16', 'LE', 'unsigned', 'Standard', '0', '1', '0', '-Inf', 'Inf'; 'LED1', '16', '16', 'LE', 'unsigned', 'Standard', '0', '1', '0', '-Inf', 'Inf'; 'LED2', '32', '8', 'LE', 'unsigned', 'Standard', '0', '1', '0', '-Inf', 'Inf' }
      settings: SourceProductName=Simulink Real-Time  SourceProductBaseCode=XP  DataFormat=manually specified signals
  CAN Setup : speedgoatlib_IO612/CAN Setup  id=1  drvLtr=C:  PCISlot=-1  port1=CAN (HS)  port2=CAN (HS)  port3=CAN (HS)  port4=Disable  opModeCAN1=Highspeed (HS)  bdrCAN1=500 kBaud  usrBdrCAN1=[10, 1, 13, 2]  stdAccMaskCAN1=[0, 0]  extAccMaskCAN1=[0, 0]  opModeCAN2=Highspeed (HS)  bdrCAN2=1 MBaud  usrBdrCAN2=[5, 1, 13, 2]  stdAccMaskCAN2=[0, 0]  extAccMaskCAN2=[0, 0]  opModeCAN3=Highspeed (HS)  bdrCAN3=500 kBaud  usrBdrCAN3=[10, 1, 13, 2]  stdAccMaskCAN3=[0, 0]  extAccMaskCAN3=[0, 0]  opModeCAN4=Highspeed (HS)  bdrCAN4=1 MBaud  usrBdrCAN4=[5, 1, 13, 2]  stdAccMaskCAN4=[0, 0]  extAccMaskCAN4=[0, 0]  initStruct=[]  termStruct=[]  protl=IO612  qtyMod=1  chNo=[1, 2, 3, 4]  ptTypes=[1, 1, 1, 1]  protlHelpIdx=[0, 1, 2, 3]  isFDMod=0
      settings: SourceProductName=Simulink Real-Time: Speedgoat Library
  CAN Write2 : speedgoatlib_IO612/CAN Write  id=1  sampleTime=0.008  portSelection=2  messageType=CAN  enaStatusPort=off  protl=IO612  ptIdx=1  isFDMod=0
      settings: SourceProductName=Simulink Real-Time: Speedgoat Library
  CAN Write5 : speedgoatlib_IO612/CAN Write  id=1  sampleTime=0.003  portSelection=1  messageType=CAN  enaStatusPort=off  protl=IO612  ptIdx=0  isFDMod=0
      settings: SourceProductName=Simulink Real-Time: Speedgoat Library
  Data Type Conversion : DataTypeConversion  OutMin=0  OutMax=65535  OutDataTypeStr=uint16  RndMeth=Nearest
  Digital IO Interface : speedgoatlib_fpga/Setup/Setup  board=IO306-25k  id=1  frontIO=None  rearIO=None  bitstreamFile=speedgoat_IO306_25k_CI_01749  rev=1.0  timestamp_string=00/00/00 00:00:00  fpgaFreq=33 MHz  fpgaTick=30.303 ns  ProgSpiFlash=off  ProgBPIFlash=off  pciSlot=-1  PullRPort0=pull-up 3.3V  VioPort0=3.3V  PullRPort1=pull-up 3.3V  VioPort1=3.3V  PullRPort2=pull-up 3.3V  VioPort2=3.3V  PullRPort3=pull-up 3.3V  VioPort3=3.3V  PullRPort4=pull-up 3.3V  VioPort4=3.3V  PullRPort5=pull-up 3.3V  VioPort5=3.3V  PullRPort6=pull-up 3.3V  VioPort6=3.3V  PullRPort15=pull-up 3.3V  PullRPort31=pull-up 3.3V  PullRPort47=pull-up 3.3V  PullRPort63=pull-up 3.3V
      settings: SourceProductName=Simulink Real-Time: Speedgoat I/O Driver Library
  Digital input : speedgoatlib_fpga_dio/Digital input  id=1  chan=[1 2]  ts=-1  pciSlot=-1  board=IO306-25k  vectorizeOutput=off
      settings: SourceProductName=Simulink Real-Time: Speedgoat Library
  Gain : Gain  Gain=2
  Gain1 : Gain  Gain=1/9
  Gain2 : Gain  Gain=1/2
  Gain6 : Gain  Gain=9
  Gain7 : Gain  Commented=on  Gain=2
  Gain8 : Gain  Commented=on  Gain=36
  Goto3 : Goto  Commented=on  GotoTag=St_spd2  TagVisibility=global
  Multiply1 : Product  Inputs=3
  Mux1 : Mux  Inputs=3
  Postion Process (double datatype) : MATLAB Function  TreatAsAtomicUnit=on
  RPM Display : Subsystem
  Rate Transition : RateTransition  Deterministic=off
  Rate Transition1 : RateTransition  Deterministic=off
  Saturation : Saturate  UpperLimit=100  LowerLimit=0
  Saturation1 : Saturate  UpperLimit=100  LowerLimit=0
  Saturation2 : Saturate  UpperLimit=100  LowerLimit=0
  Saturation3 : Saturate  UpperLimit=3.3  LowerLimit=-3.3
  Scope 3 : slrtlib/Displays and Logging/Scope   scopeno=4  scopetype=Target  autostart=off  viewmode=Graphical redraw  formatstr='%15.6f'  grid=on  ylimits=[0,0]  nosamples=3000000  noprepostsamples=0  interleave=2  triggermode=FreeRun  triggersignal=1  trigsignalfromport=off  triggerlevel=0.0  triggerslope=Either  triggerscope=1  triggersample=0  filename=YJX.yjx  mode=Lazy  writesize=512  autorestart=off  dynamicfilemode=off  maxwritefilesize=512*1024^2
  Shiftting Display : Subsystem
  Spd Dev : Subsystem
  Terminator : Terminator
  Terminator2 : Terminator
  Terminator3 : Terminator
  "Torque Switch Interface " : Subsystem
  While Iterator Subsystem : Subsystem  TreatAsAtomicUnit=on
  alpha_dis : Subsystem  TreatAsAtomicUnit=on
  loading scope : slrtlib/Displays and Logging/Scope   Commented=on  scopeno=7  scopetype=Target  autostart=on  viewmode=Graphical rolling  formatstr='%15.6f'  grid=on  ylimits=[-20,20]  nosamples=1000  noprepostsamples=0  interleave=1  triggermode=FreeRun  triggersignal=1  trigsignalfromport=off  triggerlevel=0.0  triggerslope=Either  triggerscope=1  triggersample=0  filename=data.dat  mode=Lazy  writesize=512  autorestart=off  dynamicfilemode=off  maxwritefilesize=512*1024^2
  loading scope3 : slrtlib/Displays and Logging/Scope   Commented=on  scopeno=9  scopetype=Target  autostart=on  viewmode=Graphical rolling  formatstr='%15.6f'  grid=on  ylimits=[-10,110]  nosamples=1000  noprepostsamples=0  interleave=1  triggermode=FreeRun  triggersignal=1  trigsignalfromport=off  triggerlevel=0.0  triggerslope=Either  triggerscope=1  triggersample=0  filename=data.dat  mode=Lazy  writesize=512  autorestart=off  dynamicfilemode=off  maxwritefilesize=512*1024^2
  main enable : Constant
  tag scope: IMS_torque=global, St_angle=global, St_angle_target=global, St_spd=global, St_torque=global, Switch_lamp_voltage=global, pedal_acc=global, pedal_brk=global, pedal_clt=global
  wires:
  "Analog input v2 "/1 -> [IMS_torque]
  "Analog input v2 "/2 -> Gain8/1, Gain7/1, Gain/1
  Gain/1 -> Terminator3/1
  "Analog input v2 "/3 -> Gain6/1
  [Load_motor_voltage] -> Scope 3/1, "Analog output v2 "/1
  [Switch_lamp_voltage] -> "Analog output v2 "/2
  [St_angle_corrected] -> Gain1/1
  Gain1/1 -> "Analog output v2 "/3
  [St_torque] -> Gain2/1
  Gain2/1 -> "Analog output v2 "/4
  CAN Pack3/1 -> CAN Write2/1
  Data Type Conversion/1 -> CAN Pack3/1
  Gain6/1 -> [St_angle_target]  "Steering angle target"
  Gain7/1 -> loading scope/1
  Gain8/1 -> Goto3/1
  "Analog input v2 "/4 -> 1-D Lookup Table2/1  "p_acc0"
  Saturation1/1 -> [pedal_brk]  "p_brk"
  Saturation/1 -> [pedal_clt]  "p_clt"
  [pedal_acc] -> Mux1/1
  Mux1/1 -> loading scope3/1
  [pedal_brk] -> Mux1/2
  [pedal_clt] -> Mux1/3
  "Analog input v2 "/6 -> 1-D Lookup Table/1  "p_clt"
  "Analog input v2 "/5 -> 1-D Lookup Table1/1  "p_brk0"
  Saturation2/1 -> [pedal_acc]  "p_acc"
  1-D Lookup Table/1 -> Saturation/1  "p_clt"
  1-D Lookup Table1/1 -> Saturation1/1  "p_brk"
  1-D Lookup Table2/1 -> Saturation2/1  "p_acc"
  "Torque Switch Interface "/1(Out1) -> [Switch_lamp_voltage]
  CAN Pack 1/1 -> CAN Write5/1
  Spd Dev/1(Out1) -> [St_spd]
  Multiply1/1 -> CAN Pack 1/1
  While Iterator Subsystem/1(st_angle) -> Rate Transition/1
  Rate Transition/1 -> Postion Process (double datatype)/1(pos_input)  "Steering wheel angle"
  Postion Process (double datatype)/1(pos_output) -> Spd Dev/1(In1), [St_angle]  "Steering wheel angle"
  [Assist_cmd] -> Saturation3/1
  While Iterator Subsystem/3(st_current) -> Terminator/1
  Saturation3/1 -> CAN Pack 1/2  "motor_torque"
  [Str_clrflg] -> Multiply1/2
  Rate Transition1/1 -> [St_torque]  "Steering_torque"
  main enable/1 -> Multiply1/1
  [T_switch] -> Multiply1/3
  While Iterator Subsystem/2(st_torque) -> Rate Transition1/1
  Abs/1 -> Data Type Conversion/1
  A_dis/1 -> Terminator2/1
  Shiftting Display/1(Out1) -> CAN Pack3/3
  Digital input/1 -> "Torque Switch Interface "/1(b_on)  "b_on"
  Digital input/2 -> "Torque Switch Interface "/2(b_off)  "b_off"
  [Vehicle_speed] -> Abs/1
  RPM Display/1(Out1) -> CAN Pack3/2
